simulink model "final_model"  (R2022b)
settings: Solver=VariableStepAuto  StartTime=0.0  StopTime=5  RelTol=1e-3
values from neighbouring files (symbols this model uses):
  g = 9.81    [gyro_and_bicycle_params.m]
  Ip = Ifz    (= 0.09)    [gyro_and_bicycle_params.m]
  k1 = Ibz + mb*hb^2 + mf*hf^2 + (Ifz + Ifx + 2*mf*hf^2) + mg*hg^2 +(Igz + Igx + 2*mg*hg^2)    (= 20.1934)    [gyro_and_bicycle_params.m]
  k2 = mb*hb + mf*hf + mg*hg    (= 17.89)    [gyro_and_bicycle_params.m]
  wp = 2000 * 2*pi/60    (= 209.439510239)    [gyro_and_bicycle_params.m]
libraries: slpidlib x1
settings Model: Creator=baran  LastModifiedBy=baran

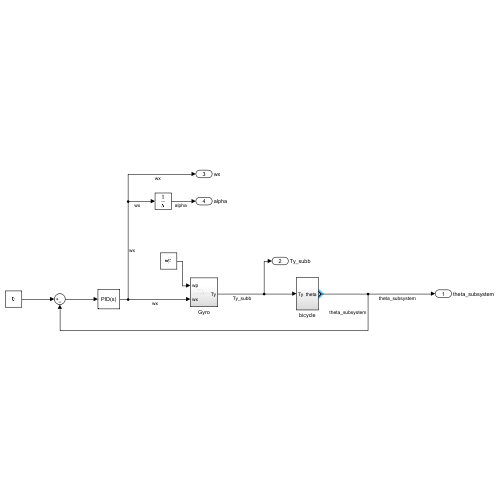
[thumbnail: Simulink's stored preview of the top-level diagram]
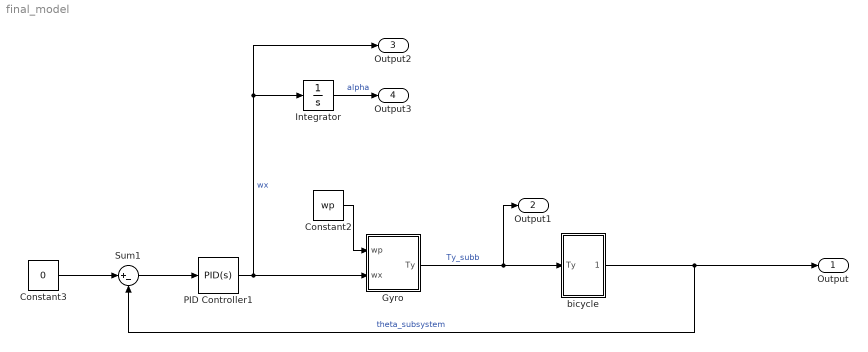
== system final_model ==
  Constant2 : Constant  Value=wp
  Constant3 : Constant  Value=0
  Gyro : Subsystem
  Integrator : Integrator
  PID Controller1 : slpidlib/PID Controller  Controller=PID  Form=Parallel  TimeDomain=Continuous-time  UseExternalTs=off  SampleTime=-1  IntegratorMethod=Forward Euler  FilterMethod=Forward Euler  ControllerParametersSource=internal  P=36.6985998517447  I=28.461523758298  UseKiTs=off  D=7.79499536669967  N=12.6270823091579  UseFilter=on  TunerSelectOption=Transfer Function Based (PID Tuner App)  InitialConditionSource=internal  InitialConditionForIntegrator=0  InitialConditionForFilter=0  DifferentiatorICPrevScaledInput=0  ExternalReset=none  TrackingMode=off  Kt=1  LimitOutput=off  SatLimitsSource=internal  UpperSaturationLimit=inf  LowerSaturationLimit=-inf  LinearizeAsGain=on  AntiWindupMode=none  Kb=1  LimitIntegrator=off  UpperIntegratorSaturationLimit=inf  LowerIntegratorSaturationLimit=-inf  POutMin=[]  POutMax=[]  IOutMin=[]  IOutMax=[]  DOutMin=[]  DOutMax=[]  NOutMin=[]  NOutMax=[]  SumOutMin=[]  SumOutMax=[]  SaturationOutMin=[]  SaturationOutMax=[]  PParamMin=[]  PParamMax=[]  IParamMin=[]  IParamMax=[]  DParamMin=[]  DParamMax=[]  NParamMin=[]  NParamMax=[]  KbParamMin=[]  KbParamMax=[]  KtParamMin=[]  KtParamMax=[]  KbOutMin=[]  KbOutMax=[]  KtOutMin=[]  KtOutMax=[]  IntegratorOutMin=[]  IntegratorOutMax=[]  FilterOutMin=[]  FilterOutMax=[]  SumI1OutMin=[]  SumI1OutMax=[]  SumI2OutMin=[]  SumI2OutMax=[]  SumI3OutMin=[]  SumI3OutMax=[]  SumI4OutMin=[]  SumI4OutMax=[]  SumDOutMin=[]  SumDOutMax=[]  DifferentiatorOutMin=[]  DifferentiatorOutMax=[]  FilterDiffOutCoefMin=[]  FilterDiffOutCoefMax=[]  ReciprocalOutMin=[]  ReciprocalOutMax=[]  SumDenOutMin=[]  SumDenOutMax=[]  SumNumOutMin=[]  SumNumOutMax=[]  DivideOutMin=[]  DivideOutMax=[]  UdiffTsProdOutMin=[]  UdiffTsProdOutMax=[]  NTsProdOutMin=[]  NTsProdOutMax=[]  UintegralTsProdOutMin=[]  UintegralTsProdOutMax=[]  UngainTsProdOutMin=[]  UngainTsProdOutMax=[]  ClampingZeroOutDataTypeStr=Inherit: Inherit via back propagation  ClampingZeroOutMin=[]  ClampingZeroOutMax=[]  FilterDenConstantOutDataTypeStr=Inherit: Inherit via back propagation  FilterDenConstantOutMin=[]  FilterDenConstantOutMax=[]  PCopyOutDataTypeStr=Inherit: Inherit via back propagation  PCopyOutMin=[]  PCopyOutMax=[]  NCopyOutDataTypeStr=Inherit: Inherit via back propagation  NCopyOutMin=[]  NCopyOutMax=[]  IntegratorContinuousStateAttributes=''  IntegratorStateMustResolveToSignalObject=off  IntegratorRTWStateStorageClass=Auto  FilterContinuousStateAttributes=''  FilterStateMustResolveToSignalObject=off  FilterRTWStateStorageClass=Auto  ParallelPVariant=InternalParameters  IdealPVariant=Disabled  IVariant=InternalParameters  DVariant=InternalParameters  IntegratorVariant=Continuous  SatVariant=Disabled  AWVariant=Passthrough  PCopyVariant=Disabled  TRVariant=Disabled  FdbkBlocksVariant=Forward  IdealPFdbkVariant=Disabled  SatFdbkVariant=Disabled  DerivativeFilterVariant=ContFilter  NVariant=InternalParameters  NCopyVariant=Disabled  FilterICVariant=InternalICsFilter  IntegratorICVariant=InternalICs  ExternalResetVariant=Disabled  TRSumVariant=Passthrough  SumFdbkVariant=Disabled  SumVariant=Sum_PID  TsampFilterVariant=InternalTs  TsampNgainVariant=Passthrough  TsampIntegralVariant=Passthrough  ExternalSaturationOutDataTypeStr=Inherit: Same as second input
  Sum1 : Sum  Inputs=|+-
  bicycle : Subsystem
  Output : Outport  SignalName=theta_subsystem
  Output1 : Outport  Port=2  SignalName=Ty_subb
  Output2 : Outport  Port=3  SignalName=wx
  Output3 : Outport  Port=4  SignalName=alpha
  wires:
  PID Controller1/1 -> Output2/1, Integrator/1, Gyro/2(wx)  "wx"
  Sum1/1 -> PID Controller1/1
  Gyro/1(Ty) -> Output1/1, bicycle/1(Ty)  "Ty_subb"
  Constant3/1 -> Sum1/1
  Constant2/1 -> Gyro/1(wp)
  bicycle/1(theta) -> Output/1, Sum1/2  "theta_subsystem"
  Integrator/1 -> Output3/1  "alpha"

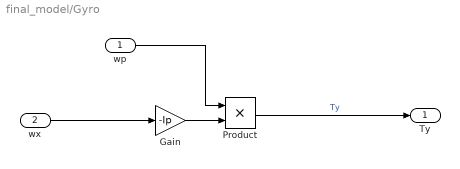
== system final_model/Gyro ==
  wp : Inport
  wx : Inport  Port=2
  Gain : Gain  Gain=-Ip
  Product : Product
  Ty : Outport
  wires:
  Gain/1 -> Product/2
  Product/1 -> Ty/1  "Ty"
  wx/1 -> Gain/1
  wp/1 -> Product/1

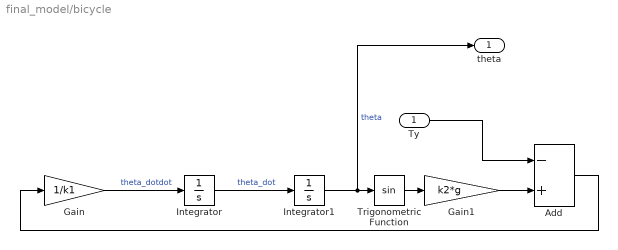
== system final_model/bicycle ==
  Ty : Inport
  Add : Sum  Inputs=-+
  Gain : Gain  Gain=1/k1
  Gain1 : Gain  Gain=k2*g
  Integrator : Integrator
  Integrator1 : Integrator  InitialCondition=-0.05
  Trigonometric Function : Trigonometry
  theta : Outport
  wires:
  Gain1/1 -> Add/2
  Integrator/1 -> Integrator1/1  "theta_dot"
  Integrator1/1 -> theta/1, Trigonometric Function/1  "theta"
  Gain/1 -> Integrator/1  "theta_dotdot"
  Ty/1 -> Add/1
  Add/1 -> Gain/1
  Trigonometric Function/1 -> Gain1/1
